simulink model "task_1_sim"  (R2022b)
settings: Solver=VariableStepAuto  StartTime=0.0  StopTime=10.0  RelTol=1e-3
model workspace (MAT data in the model file):
  C0 = [1  0  0  0  0  0; 0  1  0  0  0  0; 0  0  1  0  0  0; 0  0  0  1  0  0; 0  0  0  0  1  0; 0  0  0  0  0  1]
  D0 = [0  0; 0  0; 0  0; 0  0; 0  0; 0  0]
  input = [0 0]
values from neighbouring files (symbols this model uses):
  K1_1 = KBar*T    [task1.m]
undefined symbols (not defined in the file or in its folder): A, B, C
settings Model: Creator=小灰  LastModifiedBy=小灰

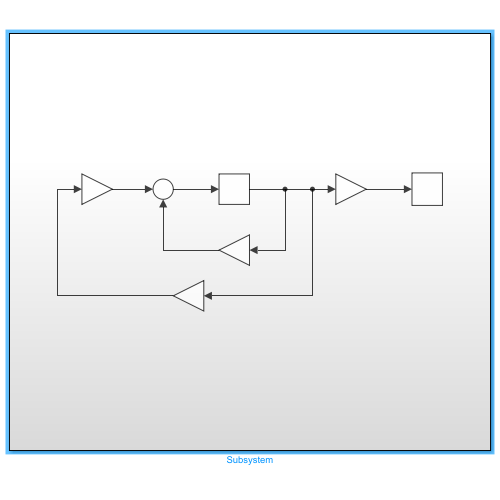
[thumbnail: Simulink's stored preview of the top-level diagram]
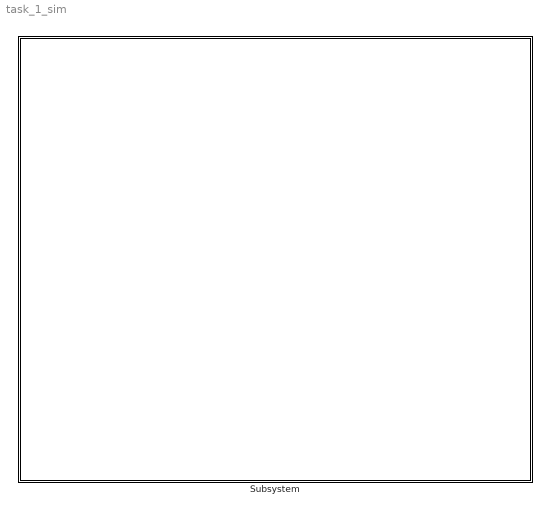
== system task_1_sim ==
  Subsystem : Subsystem

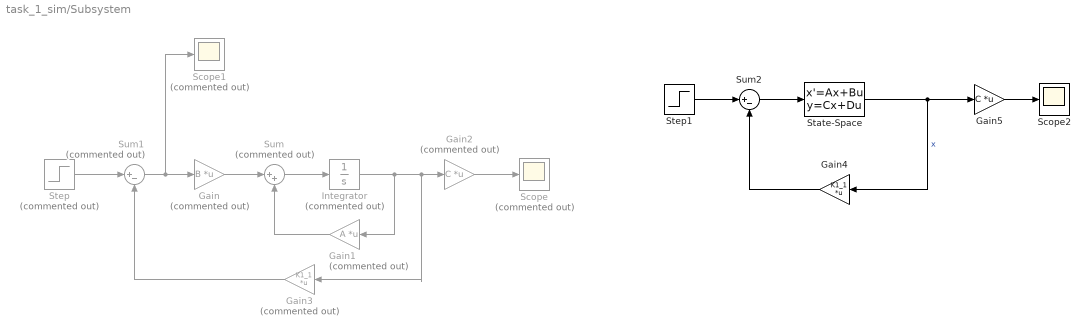
== system task_1_sim/Subsystem ==
  Gain : Gain  Commented=on  Gain=B  Multiplication=Matrix(K*u)
  Gain1 : Gain  Commented=on  Gain=A  Multiplication=Matrix(K*u)
  Gain2 : Gain  Commented=on  Gain=C  Multiplication=Matrix(K*u)
  Gain3 : Gain  Commented=on  Gain=K1_1  Multiplication=Matrix(K*u)
  Gain4 : Gain  Gain=K1_1  Multiplication=Matrix(K*u)
  Gain5 : Gain  Gain=C  Multiplication=Matrix(K*u)
  Integrator : Integrator  Commented=on
  Scope : Scope  Commented=on
  Scope1 : Scope  Commented=on
  Scope2 : Scope
  State-Space : StateSpace  A=A  B=B  C=C0  D=D0  InitialCondition=0  ParameterTunability=Unconstrained
  Step : Step  Commented=on  SampleTime=0
  Step1 : Step  Before=[0, 0]  After=[1, 0]  SampleTime=0
  Sum : Sum  Commented=on  Inputs=|++
  Sum1 : Sum  Commented=on  Inputs=|+-
  Sum2 : Sum  Inputs=|+-
  wires:
  Gain1/1 -> Sum/2
  Gain/1 -> Sum/1
  Sum/1 -> Integrator/1
  Integrator/1 -> Gain1/1, Gain3/1, Gain2/1
  Gain2/1 -> Scope/1
  Gain3/1 -> Sum1/2
  Sum1/1 -> Scope1/1, Gain/1
  Step/1 -> Sum1/1
  Step1/1 -> Sum2/1
  State-Space/1 -> Gain5/1, Gain4/1  "x"
  Sum2/1 -> State-Space/1
  Gain4/1 -> Sum2/2
  Gain5/1 -> Scope2/1
